simulink model "backup_LQR"  (R2019b)
settings: Solver=ode1  StartTime=0.0  StopTime=Inf  FixedStep=0.001  RelTol=1e-3
PostLoadFcn:
  | , if any(exist('dsrtsu_mdlpostloadfcn', 'file') ~= 0), dsrtsu_mdlpostloadfcn('Execute', bdroot); end,
InitFcn:
  | , if any(exist('rtifpga_mdlclblib', 'file') ~= 0), rtifpga_mdlclblib('Init', bdroot); end,
values from neighbouring files (symbols this model uses):
  ballLQRgain = lqr(ballSystem, Q, R)    [linear_Feedback_ball.m]
  denc_mi = Controller.Denominator{1}    [linear_Feedback_ball.m]
  numc_mi = Controller.Numerator{1}    [linear_Feedback_ball.m]
undefined symbols (not defined in the file or in its folder): Continuous, Time, Ybop0
libraries: rtiemclib x6, rtiethernetlib x3, rti1202lib_dac_class1 x3, ctrlSharedLib x1
(part 1 of 2)
Description:
  | Standard RTI1202 template.
  | Supported MATLAB version:  R2019b.
settings Model: Tag=RTI1202  DSRTSU_INTERNAL_RTI_VER=570  DSRTSU_INTERNAL_RTI_TYPE=rti1202  RTICANMMDATA=struct('GeneralSetupData',struct('modelroot','C:\Users\20200910\Documents\Temp\14062021','generalsettings',struct('filesettings',struct('destfolder',struct('Name','RTICANMM_FILES','Check',1),'buildfolder',struct('Name','.','Check',1),'AbsDestfolder',struct('Name','C:\Users\20200910\Documents\Temp\14062021\RTICANMM_FILES'),'AbsBuildfolder',struct('Name','C:\Users\20200910\Documents\Temp\14062021'))),'options',struct('addpaths',1,'rmpaths',1,'addtrcexclusion',true,'cannavigator',struct('checkmonitoring',0),'show_usrtrc',0,'use_usrtrc',0),'advanced',struct('options',ones(1,100)),'MPSetup',{{}},'RTI',struct('Type','RTI1202','Ver','7.15','Date','02-Nov-2020'),'modelname','backup_LQR','block','backup_LQR'))  DSRTSU_INTERNAL_RTIFPGA=170  Creator=20201603  LastModifiedBy=20200910
settings DataIOCC: ReturnWorkspaceOutputs=off
settings OptimizationCC: BlockReduction=off  OptimizeBlockIOStorage=off  BufferReuse=off  GlobalBufferReuse=off  ExpressionFolding=off  LocalBlockOutputs=off  OptimizeDataStoreBuffers=off  BusAssignmentInplaceUpdate=off
settings DebuggingCC: PregeneratedLibrarySubsystemCodeDiagnostic=none  ArithmeticOperatorsInVariantConditions=warning
settings HardwareCC: ProdBitPerPointer=32  ProdBitPerSizeT=32  ProdBitPerPtrDiffT=32  ProdLargestAtomicInteger=Integer  ProdEndianess=BigEndian  ProdWordSize=32  ProdLongLongMode=on  ProdHWDeviceType=Custom Processor->Custom  TargetIntDivRoundTo=Zero  TargetEndianess=BigEndian  TargetHWDeviceType=Custom Processor->Custom
settings ModelReferenceCC: EnableParallelModelReferenceBuilds=on  ParallelModelReferenceMATLABWorkerInit=Load Top Model
settings SFSimCC: SimUseLocalCustomCode=off  MATLABDynamicMemAlloc=off  CustomCodeUndefinedFunction=UseInterfaceOnly
settings RTWCC: Description=dSPACE DS1202 Hardware Platform  SystemTargetFile=rti1202.tlc  MakeCommand=make_rti  TemplateMakefile=rti1202.tmf  RTWUseLocalCustomCode=off
settings CodeAppCC: StateflowObjectComments=on
settings STFCustomTargetCC: ParMdlRefBuildCompliant=on  SystemTargetFile=rti1202.tlc
settings GRTTargetCC: TargetLangStandard=C89/C90 (ANSI)  CompOptLevelCompliant=off  ConcurrentExecutionCompliant=off  CombineOutputUpdateFcns=off  MatFileLogging=off  CPPClassGenCompliant=off  UseToolchainInfoCompliant=off
settings ConfigComp: CovMetricSettings=dswe

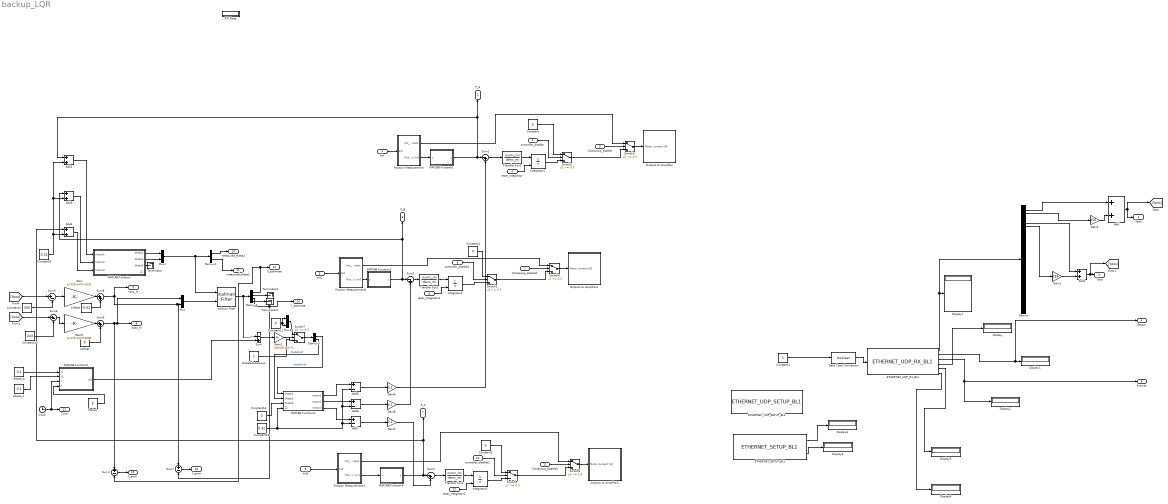
== system backup_LQR ==
  Init : Inport
  controller_disable : Inport  Port=2
  CloseLoop_disable : Inport  Port=3
  reser_integrator : Inport  Port=4
  Init1 : Inport  Port=5
  controller_disable1 : Inport  Port=6
  CloseLoop_disable1 : Inport  Port=7
  reser_integrator1 : Inport  Port=8
  Init2 : Inport  Port=9
  controller_disable2 : Inport  Port=10
  CloseLoop_disable2 : Inport  Port=11
  reser_integrator2 : Inport  Port=12
  Add : Sum  AccumDataTypeStr=uint16
  Add{1..4} (4 alike) : Sum
  Add5 : Sum  Inputs=+-
  Add6 : Sum  Inputs=+-
  Add7 : Sum  Inputs=+-
  Clock : Clock
  Constant{,2..3,11,13} (5 alike) : Constant  Value=0
  Constant1 : Constant
  Constant10 : Constant  Value=243
  Constant14 : Constant  Value=0.32
  Constant4 : Constant  Value=300
  Constant9 : Constant  Value=0.32
  Data Type Conversion : DataTypeConversion  OutDataTypeStr=boolean
  Demux : Demux  Outputs=32
  Demux1 : Demux  Outputs=2
  Demux2 : Demux
  Demux3 : Demux  Outputs=2
  "DisableOuterLoop " : Constant
  Display{,1..7} (8 alike) : Display
      Display7 settings: Format=decimal (Stored Integer)
  ETHERNET_SETUP_BL1 : rtiethernetlib/ETHERNET_SETUP_BL1  DSProperties=struct('RTI',struct('Version',uint32(2),'BlockType',struct('isSLSource',uint8(0),'isSLSink',uint8(0),'isHWSource',uint8(0),'isHWSink',uint8(0),'isSetup',uint8(1),'isInline',uint8(1),'isNonInline',uint8(0),'isInterrupt',uint8(0),'isChannelwise',uint8(0)),'IOBoardType','DSETHERNET','UnitType','ETHERNET','Identifier','SETUP','DialogType','ML','BlockSet','RTIETHERNET','SlaveProcessor','NONE'))  RTIBlockInterface=struct('OutputPortsWidth',int32([3 1 1 4]),'OutputPortsActive',[1 0 0 1],'OutputPortsName',{{['Link Status'],['Watchdog Status'],['DHCP Status'],['Local IP']}},'OutputPortsDataType',{{'SS_UINT32','SS_UINT32','SS_UINT32','SS_UINT8'}},'InitLevel',3,'IconTransparency','on','BlockDisplay',{{['Ethernet Setup\n\nLocal IP: 192.168.141.7'],'left'}},'DialogFcn','rtiethernetsetupgui','BlockName',struct('Token',{{'ETHERNET_SETUP_BL1'}}))  RTIBlockParameters=struct('DHCPserverMode',{{0,'OFF',[0 1]}},'LocalIpNum1',{{'192','OFF',[0 255]}},'LocalIpNum2',{{'168','OFF',[0 255]}},'LocalIpNum3',{{'141','OFF',[0 255]}},'LocalIpNum4',{{'7','OFF',[0 255]}},'SubnetMaskNum1',{{'255','OFF',[0 255]}},'SubnetMaskNum2',{{'255','OFF',[0 255]}},'SubnetMaskNum3',{{'255','OFF',[0 255]}},'SubnetMaskNum4',{{'0','OFF',[0 255]}},'GatewayNum1',{{'0','OFF',[0 255]}},'GatewayNum2',{{'0','OFF',[0 255]}},'GatewayNum3',{{'0','OFF',[0 255]}},'GatewayNum4',{{'0','OFF',[0 255]}},'LinkStatusOutPortMode',{{1,'OFF',[0 1]}},'NumOfEthConnectors',{{3,'ON',[1 16]}},'WatchdogStatusOutPortMode',{{0,'OFF',[0 1]}},'LocalIpOutPortMode',{{1,'OFF',[0 1]}},'IpAndSubmaskCheck',{{int32(1),'OFF',[0 1]}},'TLCFileName',{{'rtiethernetsetup','OFF',[]}})  RTISFcnParameters=struct('DHCPserverMode','int32','LocalIpNum1','uint8','LocalIpNum2','uint8','LocalIpNum3','uint8','LocalIpNum4','uint8','SubnetMaskNum1','uint8','SubnetMaskNum2','uint8','SubnetMaskNum3','uint8','SubnetMaskNum4','uint8','GatewayNum1','uint8','GatewayNum2','uint8','GatewayNum3','uint8','GatewayNum4','uint8','LinkStatusOutPortMode','int32','NumOfEthConnectors','int32','WatchdogStatusOutPortMode','int32','LocalIpOutPortMode','int32','TLCFileName','char')  RTIBlockParaDefault=struct('DHCPserverMode',0,'LocalIpNum1',192,'LocalIpNum2',168,'LocalIpNum3',140,'LocalIpNum4',6,'SubnetMaskNum1',255,'SubnetMaskNum2',255,'SubnetMaskNum3',255,'SubnetMaskNum4',0,'GatewayNum1',0,'GatewayNum2',0,'GatewayNum3',0,'GatewayNum4',0,'LinkStatusOutPortMode',1,'NumOfEthConnectors',3,'WatchdogStatusOutPortMode',0,'LocalIpOutPortMode',0,'IpAndSubmaskCheck',1,'TLCFileName','rtiethernetsetup')
      settings: SourceProductName=dSPACE RTI Ethernet Blockset
  ETHERNET_UDP_RX_BL1 : rtiethernetlib/ETHERNET_UDP_RX_BL1  DSProperties=struct('RTI',struct('Version',uint32(1),'BlockType',struct('isSLSource',uint8(1),'isSLSink',uint8(1),'isHWSource',uint8(0),'isHWSink',uint8(1),'isSetup',uint8(0),'isInline',uint8(1),'isNonInline',uint8(0),'isInterrupt',uint8(0),'isChannelwise',uint8(0)),'IOBoardType','DSETHERNET','UnitType','UDP','Identifier','RXUDP','DialogType','ML','BlockSet','RTIETHERNET','SlaveProcessor','NONE'))  RTIBlockInterface=struct('OutputPortsWidth',int32([32 1 1 1 4 1]),'OutputPortsActive',[1 1 1 1 1 1],'OutputPortsName',{{'Data','Status',['Received Frames'],['Received Bytes'],['Remote IP'],['Remote Port']}},'OutputPortsDataType',{{'SS_UINT8','SS_UINT32','SS_DOUBLE','SS_UINT32','SS_UINT8','SS_UINT16'}},'InputPortsWidth',int32(1),'InputPortsActive',1,'InputPortsName',{{'Enable'}},'InputPortsDataType',{{'SS_BOOLEAN'}},'RWork',{{{'RECEIVED_FRAMES',uint32(1)}}},'InitLevel',3,'IconTransparency','on','BlockDisplay',{{['Ethernet UDP/IP\nRX\n\nSocket ID: 0'],'center'}},'DialogFcn','rtiethernetrxudpgui','BlockName',struct('Token',{{'ETHERNET_UDP_RX_BL1'}}))  RTIBlockParameters=struct('SocketIdIndex',{{2,'OFF',[1 2]}},'SocketId',{{0,'OFF',[-1 inf]}},'RemoteIp',{{['<NOT AVAILABLE>'],'OFF',[]}},'RemotePort',{{['<NOT AVAILABLE>'],'OFF',[]}},'LocalPort',{{49001,'OFF',[]}},'FrameSize',{{'32','OFF',[1 65507]}},'EnableVariableFrameSize',{{1,'OFF',[0 1]}},'VariableFrameSizeMode',{{1,'OFF',[1 2]}},'InterruptMode',{{0,'OFF',[0 1]}},'RemoteIpOutPortMode',{{1,'OFF',[0 1]}},'RemotePortOutPortMode',{{1,'OFF',[0 1]}},'TLCFileName',{{'rtiethernetrxudp','OFF',[]}})  RTISFcnParameters=struct('SocketIdIndex','int32','SocketId','double','FrameSize','uint16','EnableVariableFrameSize','int32','VariableFrameSizeMode','int32','InterruptMode','int32','RemoteIpOutPortMode','int32','RemotePortOutPortMode','int32','TLCFileName','char')  RTIBlockParaDefault=struct('SocketIdIndex',1,'SocketId',-1,'RemoteIp',['<NOT AVAILABLE>'],'RemotePort',['<NOT AVAILABLE>'],'LocalPort',['<NOT AVAILABLE>'],'FrameSize',1024,'EnableVariableFrameSize',0,'VariableFrameSizeMode',1,'InterruptMode',0,'RemoteIpOutPortMode',0,'RemotePortOutPortMode',0,'TLCFileName','rtiethernetrxudp')
      settings: SourceProductName=dSPACE RTI Ethernet Blockset
  ETHERNET_UDP_SETUP_BL1 : rtiethernetlib/ETHERNET_UDP_SETUP_BL1  DSProperties=struct('RTI',struct('Version',uint32(2),'BlockType',struct('isSLSource',uint8(1),'isSLSink',uint8(1),'isHWSource',uint8(0),'isHWSink',uint8(0),'isSetup',uint8(0),'isInline',uint8(1),'isNonInline',uint8(0),'isInterrupt',uint8(0),'isChannelwise',uint8(0)),'IOBoardType','DSETHERNET','UnitType','UDP','Identifier','SETUPUDP','DialogType','ML','BlockSet','RTIETHERNET','SlaveProcessor','NONE'))  RTIBlockInterface=struct('OutputPortsWidth',int32(2),'OutputPortsActive',0,'OutputPortsName',{{['RX Dropped Frames']}},'OutputPortsDataType',{{'SS_DOUBLE'}},'InputPortsWidth',int32([4 1]),'InputPortsActive',int32([0 0]),'InputPortsName',{{['RX Remote IP Filter'],['RX Remote Port Filter']}},'InputPortsDataType',{{'SS_UINT8','SS_UINT16'}},'RWork',{{{'RX_DROPPED_FRAMES',uint32(2)}}},'InitLevel',3,'IconTransparency','on','BlockDisplay',{{['Ethernet UDP/IP\nSetup\n\nSocket ID: 0'],'center'}},'DialogFcn','rtiethernetsetupudpgui','BlockName',struct('Token',{{'ETHERNET_UDP_SETUP_BL1'}}))  RTIBlockParameters=struct('SocketId',{{0,'OFF',[]}},'EnableSocketBind',{{1,'OFF',[0 1]}},'AcceptAnyRxRemoteIp',{{1,'OFF',[0 1]}},'RxRemoteIpNum1',{{'131','OFF',[0 255]}},'RxRemoteIpNum2',{{'155','OFF',[0 255]}},'RxRemoteIpNum3',{{'33','OFF',[0 255]}},'RxRemoteIpNum4',{{'44','OFF',[0 255]}},'EnableDynamicRxRemoteIpFilter',{{0,'OFF',[0 1]}},'AcceptAnyRxRemotePort',{{1,'OFF',[0 1]}},'RxRemotePort',{{'57272','OFF',[1 65535]}},'EnableDynamicRxRemotePortFilter',{{0,'OFF',[0 1]}},'TxRemoteIpNum1',{{'131','OFF',[0 255]}},'TxRemoteIpNum2',{{'155','OFF',[0 255]}},'TxRemoteIpNum3',{{'33','OFF',[0 255]}},'TxRemoteIpNum4',{{'44','OFF',[0 255]}},'TxRemotePort',{{'49002','OFF',[1 65535]}},'SpecifyLocalPort',{{1,'OFF',[0 1]}},'LocalPort',{{'49001','OFF',[1 65535]}},'InterruptMode',{{0,'OFF',[0 1]}},'RxDroppedFramesOutPortMode',{{0,'OFF',[0 1]}},'RemoteIpNumCheck',{{0,'OFF',[0 1]}},'RemotePortCheck',{{0,'OFF',[0 1]}},'LocalPortCheck',{{1,'OFF',[0 1]}},'DHCPserverModeEnabled',{{0,'OFF',[0 1]}},'TLCFileName',{{'rtiethernetsetupudp','OFF',[]}})  RTISFcnParameters=struct('SocketId','double','EnableSocketBind','int32','AcceptAnyRxRemoteIp','int32','RxRemoteIpNum1','uint8','RxRemoteIpNum2','uint8','RxRemoteIpNum3','uint8','RxRemoteIpNum4','uint8','EnableDynamicRxRemoteIpFilter','int32','AcceptAnyRxRemotePort','int32','RxRemotePort','uint16','EnableDynamicRxRemotePortFilter','int32','TxRemoteIpNum1','uint8','TxRemoteIpNum2','uint8','TxRemoteIpNum3','uint8','TxRemoteIpNum4','uint8','TxRemotePort','uint16','SpecifyLocalPort','int32','LocalPort','uint16','InterruptMode','int32','RxDroppedFramesOutPortMode','int32','DHCPserverModeEnabled','int32','TLCFileName','char')  RTIBlockParaDefault=struct('SocketId',-1,'EnableSocketBind',1,'AcceptAnyRxRemoteIp',1,'RxRemoteIpNum1',0,'RxRemoteIpNum2',0,'RxRemoteIpNum3',0,'RxRemoteIpNum4',0,'EnableDynamicRxRemoteIpFilter',0,'AcceptAnyRxRemotePort',1,'RxRemotePort',49002,'EnableDynamicRxRemotePortFilter',0,'TxRemoteIpNum1',0,'TxRemoteIpNum2',0,'TxRemoteIpNum3',0,'TxRemoteIpNum4',0,'TxRemotePort',49002,'SpecifyLocalPort',0,'LocalPort',49001,'InterruptMode',0,'RxDroppedFramesOutPortMode',0,'RemoteIpNumCheck',0,'RemotePortCheck',0,'LocalPortCheck',0,'DHCPserverModeEnabled',0,'TLCFileName','rtiethernetsetupudp')
      settings: SourceProductName=dSPACE RTI Ethernet Blockset
  Gain : Gain  Gain=1/(536-54)*0.3595
  Gain1 : Gain  Gain=256  OutDataTypeStr=uint16
  Gain2 : Gain  Gain=256  OutDataTypeStr=uint16
  Gain3 : Gain  Gain=ballLQRgain  Multiplication=Matrix(K*u)
  Gain5 : Gain  Gain=1/(475-14)*0.3595
  GainA : Gain  Gain=0.1
  GainB : Gain  Gain=0.1
  GainC : Gain  Gain=0.1
  Integrator1 : Integrator  ExternalReset=rising  LimitOutput=on  UpperSaturationLimit=3  LowerSaturationLimit=-3
  Integrator2 : Integrator  ExternalReset=rising  LimitOutput=on  UpperSaturationLimit=3  LowerSaturationLimit=-3
  Integrator3 : Integrator  ExternalReset=rising  LimitOutput=on  UpperSaturationLimit=3  LowerSaturationLimit=-3
  Kalman Filter : ctrlSharedLib/Kalman Filter  TimeDomain=Continuous-Time  UseCurrentEstimator=on  ModelSource=LTI State-Space Variable  ModelSourceVariable=ballSystem  A=0.95  B=1  C=1  D=0  NumberOfStates=1  NumberOfInputs=1  NumberOfOutputs=1  InitialEstimateSource=Dialog  X0=Ybop0  P0=10  UseK=off  UseGH=off  NumberOfProcessNoiseInputs=1  G=1  TimeInvariantG=on  H=0  TimeInvariantH=on  Q=diag([1 20 1 20])  TimeInvariantQ=on  R=diag([0.01 0.01])  TimeInvariantR=on  N=0  TimeInvariantN=on  AddInputPort=on  AddEnablePort=off  OutputEstimatedY=off  OutputP=off  Ts=-1
      settings: SourceProductBaseCode=CT
  MATLAB Function : MATLAB Function  TreatAsAtomicUnit=on
  MATLAB Function1 : MATLAB Function  TreatAsAtomicUnit=on
  MATLAB Function2 : MATLAB Function  TreatAsAtomicUnit=on
  MATLAB Function3 : MATLAB Function  TreatAsAtomicUnit=on
  MATLAB Function4 : MATLAB Function  TreatAsAtomicUnit=on
  MATLAB Function5 : MATLAB Function  TreatAsAtomicUnit=on
  Mux : Mux  Inputs=2
  Mux1 : Mux  Inputs=2
  Mux4 : Mux  Inputs=2
  Outputs to Amplifier : Subsystem  TreatAsAtomicUnit=on
  Outputs to Amplifier1 : Subsystem  TreatAsAtomicUnit=on
  Outputs to Amplifier2 : Subsystem  TreatAsAtomicUnit=on
  Period : Constant  Value=5
  Position Measurement : Subsystem  TreatAsAtomicUnit=on
  Position Measurement1 : Subsystem  TreatAsAtomicUnit=on
  Position Measurement2 : Subsystem  TreatAsAtomicUnit=on
  RTI Data : Subsystem  Tag=struct('RTIDataServer',struct('RTIDataServerVs','2','RTIModelDescription','struct(''main'',''backup_LQR'',''sub'','''',''isMp'',0)'))  LoadFcn="if exist('rtidc'), try,  rtidc('DataHostBlockClbLoad', gcbh); catch, disp(['Warning: ''LoadFcn'' for RTI Data block failed: ' lasterr]); end, end,"  mask(RTI_DATA_HOST){}
      mask help:
      | RTI Data Block.
      | This block is used by RTI to store internal model-dependent data.
      | Please keep this block on the root level of the model. Deleting this block will result in data loss.
      |
      | NEVER DELETE OR COPY THIS BLOCK!
      settings: CopyFcn="if exist('rtidc'), try,  rtidc('DataHostBlockClbCopy', gcbh); catch, disp(['Warning: ''CopyFcn'' for RTI Data block failed: ' lasterr]); end, end,"  DeleteFcn="if exist('rtidc'), try,  rtidc('DataHostBlockClbDelete', gcbh); catch, disp(['Warning: ''DeleteFcn'' for RTI Data block failed: ' lasterr]); end, end,"  ModelCloseFcn="if exist('rtidc'), try,  rtidc('DataHostBlockClbModelClose', gcbh); catch, disp(['Warning: ''ModelCloseFcn'' for RTI Data block failed: ' lasterr]); end, end,"  PreSaveFcn="if exist('rtidc'), try,  rtidc('DataHostBlockClbPreSave', gcbh); catch, disp(['Warning: ''PreSaveFcn'' for RTI Data block failed: ' lasterr]); end, end,"  PostSaveFcn="if exist('rtidc'), try,  rtidc('DataHostBlockClbPostSave', gcbh); catch, disp(['Warning: ''PostSaveFcn'' for RTI Data block failed: ' lasterr]); end, end,"  NameChangeFcn="if exist('rtidc'), try,  rtidc('DataHostBlockClbNameChange', gcbh); catch, disp(['Warning: ''NameChangeFcn'' for RTI Data block failed: ' lasterr]); end, end,"
      mask Help:
      | RTI Data Block.
      | This block is used by RTI to store internal model-dependent data.
      | Please keep this block on the root level of the model. Deleting this block will result in data loss.
      | 
      | NEVER DELETE OR COPY THIS BLOCK!
      mask Display:
      | text(0.5, 0.5, 'RTI Data', 'HorizontalAlignment', 'center');
      | plot([1 0]);
  Sum : Sum  Inputs=|-+
  Sum1 : Sum  Inputs=|-+  SaturateOnIntegerOverflow=on
  Sum2 : Sum  Inputs=|-+  SaturateOnIntegerOverflow=on
  Sum3 : Sum  Inputs=|-+  SaturateOnIntegerOverflow=on
  Sum4 : Sum  Inputs=+-
  Sum5 : Sum  Inputs=|+-
  Sum6 : Sum  Inputs=|+-
  Sum7 : Sum  Inputs=+-
  Sum8 : Sum  Inputs=|++
  Sum9 : Sum  Inputs=|++
  Switch{1..7} (7 alike) : Switch  Threshold=0.5
  Terminator : Terminator
  Terminator1 : Terminator
  Terminator2 : Terminator
  Transfer Fcn1 : TransferFcn  Numerator=numc_mi  Denominator=denc_mi
  Transfer Fcn2 : TransferFcn  Numerator=numc_mi  Denominator=denc_mi
  Transfer Fcn3 : TransferFcn  Numerator=numc_mi  Denominator=denc_mi
  Xoffset : Constant  Value=0
  Yoffset : Constant  Value=-0.02
  ellipse_a : Constant  Value=0.1
  ellipse_b : Constant  Value=0.1
  P_A : Outport
  "Xpos " : Outport  Port=2
  "Ypos " : Outport  Port=3
  "Status " : Outport  Port=4
  "Frames " : Outport  Port=5
  P_B : Outport  Port=6
  P_C : Outport  Port=7
  Xpos_m : Outport  Port=8
  Ypos_m : Outport  Port=9
  measured_theta1 : Outport  Port=10
  measured_theta2 : Outport  Port=11
  Time : Outport  Port=12
  X_estimate : Outport  Port=13
  Y_estimate : Outport  Port=14
  X_error : Outport  Port=15
  Y_error : Outport  Port=16
  wires:
  Add5/1 -> GainA/1
  reser_integrator/1 -> Integrator2/2
  controller_disable/1 -> Switch2/2
  CloseLoop_disable/1 -> Switch3/2
  Position Measurement/1(init_current) -> Switch3/1
  Init/1 -> Position Measurement/1(Init)
  Constant/1 -> Switch2/1
  Switch3/1 -> Outputs to Amplifier/1(Motor current [A])
  Switch2/1 -> Switch3/3
  Gain2/1 -> Add/2
  Demux/1 -> Add/1
  Add1/1 -> [Ypos], "Ypos "/1
  ETHERNET_SETUP_BL1/2 -> Display3/1
  Demux/2 -> Gain2/1
  ETHERNET_UDP_RX_BL1/2 -> "Status "/1, Display1/1
  ETHERNET_UDP_RX_BL1/6 -> Display4/1
  Demux/5 -> Add1/1
  ETHERNET_UDP_RX_BL1/4 -> Display/1
  Data Type Conversion/1 -> ETHERNET_UDP_RX_BL1/1
  ETHERNET_UDP_RX_BL1/3 -> "Frames "/1, Display2/1
  Constant1/1 -> Data Type Conversion/1
  Add/1 -> "Xpos "/1, [Xpos]
  Gain1/1 -> Add1/2
  Demux/6 -> Gain1/1
  ETHERNET_SETUP_BL1/1 -> Display6/1
  ETHERNET_UDP_RX_BL1/1 -> Display7/1, Demux/1
  ETHERNET_UDP_RX_BL1/5 -> Display5/1
  CloseLoop_disable1/1 -> Switch4/2
  Init1/1 -> Position Measurement1/1(Init)
  Add6/1 -> GainB/1
  controller_disable1/1 -> Switch1/2
  reser_integrator1/1 -> Integrator1/2
  MATLAB Function2/1(y) -> Add3/1, P_B/1, Sum2/1
  Switch4/1 -> Outputs to Amplifier1/1(Motor current [A])
  Constant2/1 -> Switch1/1
  Position Measurement1/1(init_current) -> Switch4/1
  Switch1/1 -> Switch4/3
  Constant3/1 -> Switch5/1
  controller_disable2/1 -> Switch5/2
  CloseLoop_disable2/1 -> Switch6/2
  Init2/1 -> Position Measurement2/1(Init)
  reser_integrator2/1 -> Integrator3/2
  Position Measurement2/1(init_current) -> Switch6/1
  Switch6/1 -> Outputs to Amplifier2/1(Motor current [A])
  Switch5/1 -> Switch6/3
  MATLAB Function4/1(y) -> P_C/1, Add4/1, Sum3/1
  Sum6/1 -> Gain5/1
  MATLAB Function1/1(y) -> P_A/1, Add2/1, Sum1/1
  Sum5/1 -> Gain/1
  MATLAB Function/3(theta3) -> Terminator/1
  Constant10/1 -> Sum6/2
  Add2/1 -> MATLAB Function/1(motor1)
  MATLAB Function/1(theta1) -> Mux1/1
  Constant9/1 -> Add4/2, Add3/2, Add2/2
  Add3/1 -> MATLAB Function/2(motor2)
  Constant4/1 -> Sum5/2
  Sum8/1 -> Sum7/1, Mux/2, Ypos_m/1
  [Xpos] -> Sum5/1
  Add4/1 -> MATLAB Function/3(motor3)
  [Ypos] -> Sum6/1
  MATLAB Function/2(theta2) -> Mux1/2
  Constant13/1 -> MATLAB Function3/3(theta3)
  MATLAB Function3/1(motor1) -> Add5/1
  MATLAB Function3/2(motor2) -> Add6/1
  MATLAB Function3/3(motor3) -> Add7/1
  Constant14/1 -> MATLAB Function3/4(Zc), Add7/2, Add6/2, Add5/2
  GainA/1 -> Sum1/2
  GainB/1 -> Sum2/2
  Add7/1 -> GainC/1
  Mux1/1 -> Kalman Filter/1, Demux1/1
  Demux3/1 -> MATLAB Function3/1(theta1)  "theta1ref"
  Demux3/2 -> MATLAB Function3/2(theta2)  "theta2ref"
  MATLAB Function5/1(ref) -> Sum/2
  Kalman Filter/1 -> Sum/1, Demux2/1
  Sum/1 -> Gain3/1
  Mux/1 -> Kalman Filter/2
  Demux1/1 -> measured_theta1/1
  Demux1/2 -> measured_theta2/1
  Position Measurement/2(Position [m]) -> MATLAB Function1/1(u)
  Position Measurement1/2(Position [m]) -> MATLAB Function2/1(u)
  Position Measurement2/2(Position [m]) -> MATLAB Function4/1(u)
  Sum9/1 -> Xpos_m/1, Mux/1, Sum4/1
  Integrator2/1 -> Switch2/3
  Integrator1/1 -> Switch1/3
  Integrator3/1 -> Switch5/3
  Sum3/1 -> Transfer Fcn3/1
  Sum2/1 -> Transfer Fcn1/1
  Transfer Fcn1/1 -> Integrator1/1
  Sum1/1 -> Transfer Fcn2/1
  Transfer Fcn2/1 -> Integrator2/1
  Transfer Fcn3/1 -> Integrator3/1
  Constant11/1 -> Mux4/1, Mux4/2
  Mux4/1 -> Switch7/1
  "DisableOuterLoop "/1 -> Switch7/2
  Gain3/1 -> Switch7/3
  Switch7/1 -> Demux3/1
  GainC/1 -> Sum3/2
  Clock/1 -> MATLAB Function5/3(t), Time/1
  Demux2/1 -> X_estimate/1, Sum4/2
  Demux2/3 -> Sum7/2, Y_estimate/1
  Demux2/2 -> Terminator1/1
  Demux2/4 -> Terminator2/1
  Sum4/1 -> X_error/1
  Sum7/1 -> Y_error/1
  ellipse_a/1 -> MATLAB Function5/1(r1)
  ellipse_b/1 -> MATLAB Function5/2(r2)
  Period/1 -> MATLAB Function5/4(T)
  Gain/1 -> Sum8/1
  Yoffset/1 -> Sum8/2
  Gain5/1 -> Sum9/1
  Xoffset/1 -> Sum9/2

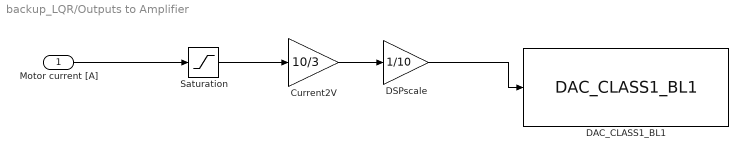
== system backup_LQR/Outputs to Amplifier ==
  Motor current [A] : Inport
  Current2V : Gain  Gain=10/3  SaturateOnIntegerOverflow=on  OutDataTypeStr=Inherit: Same as input  ParamDataTypeStr=Inherit: Same as input
  DAC_CLASS1_BL1 : rti1202lib_dac_class1/DAC_CLASS1_BL1  DSProperties=struct('RTI',struct('Version',uint32(2),'BlockType',struct('isSLSource',uint8(0),'isSLSink',uint8(1),'isHWSource',uint8(0),'isHWSink',uint8(1),'isSetup',uint8(0),'isInline',uint8(1),'isNonInline',uint8(0),'isInterrupt',uint8(0),'isChannelwise',uint8(1)),'IOBoardType',{{'DS120X','STD','DACC1'}},'UnitType','DAC','Identifier','DAC','DialogType','ML','BlockSet','NONE','SlaveProcessor','NONE'))  RTIBlockInterface=struct('InputPortsActive',1,'InputPortsWidth',int32(1),'InputPortsDataType',{{'SS_DOUBLE'}},'InputPortsName',{{['DAC 1']}},'DialogFcn','rti120xstddacc1dacgui','InitLevel',3,'IconTransparency','on','BlockDisplay',{{['DAC CL1\nChannel: 1'],'center'}},'BlockName',struct('Token',{{'DAC_CLASS1_BL1'}}))  RTIBlockParameters=struct('ChannelNo',{{1,'OFF',[]}},'ChannelNumOf',{{1,'OFF',[]}},'InitialValue1',{{'0','OFF',[-10 10]}},'InitialValue2',{{'0','OFF',[-10 10]}},'InitialValue3',{{'0','OFF',[-10 10]}},'InitialValue4',{{'0','OFF',[-10 10]}},'InitialValue5',{{'0','OFF',[-10 10]}},'InitialValue6',{{'0','OFF',[-10 10]}},'InitialValue7',{{'0','OFF',[-10 10]}},'InitialValue8',{{'0','OFF',[-10 10]}},'InitialValue9',{{'0','OFF',[-10 10]}},'InitialValue10',{{'0','OFF',[-10 10]}},'InitialValue11',{{'0','OFF',[-10 10]}},'InitialValue12',{{'0','OFF',[-10 10]}},'InitialValue13',{{'0','OFF',[-10 10]}},'InitialValue14',{{'0','OFF',[-10 10]}},'InitialValue15',{{'0','OFF',[-10 10]}},'InitialValue16',{{'0','OFF',[-10 10]}},'OutputMode',{{ones(1,16),'OFF',[1 2]}},'TermValue1',{{'0','OFF',[-10 10]}},'TermValue2',{{'0','OFF',[-10 10]}},'TermValue3',{{'0','OFF',[-10 10]}},'TermValue4',{{'0','OFF',[-10 10]}},'TermValue5',{{'0','OFF',[-10 10]}},'TermValue6',{{'0','OFF',[-10 10]}},'TermValue7',{{'0','OFF',[-10 10]}},'TermValue8',{{'0','OFF',[-10 10]}},'TermValue9',{{'0','OFF',[-10 10]}},'TermValue10',{{'0','OFF',[-10 10]}},'TermValue11',{{'0','OFF',[-10 10]}},'TermValue12',{{'0','OFF',[-10 10]}},'TermValue13',{{'0','OFF',[-10 10]}},'TermValue14',{{'0','OFF',[-10 10]}},'TermValue15',{{'0','OFF',[-10 10]}},'TermValue16',{{'0','OFF',[-10 10]}},'EnableTermMode',{{0,'OFF',[0 1]}},'TLCFileName',{{'rti120xdac_c1_dac','OFF',[]}},'InitialValueBuildCheck1',{{1,'OFF',[]}},'InitialValueBuildCheck2',{{0,'OFF',[]}},'InitialValueBuildCheck3',{{0,'OFF',[]}},'InitialValueBuildCheck4',{{0,'OFF',[]}},'InitialValueBuildCheck5',{{0,'OFF',[]}},'InitialValueBuildCheck6',{{0,'OFF',[]}},'InitialValueBuildCheck7',{{0,'OFF',[]}},'InitialValueBuildCheck8',{{0,'OFF',[]}},'InitialValueBuildCheck9',{{0,'OFF',[]}},'InitialValueBuildCheck10',{{0,'OFF',[]}},'InitialValueBuildCheck11',{{0,'OFF',[]}},'InitialValueBuildCheck12',{{0,'OFF',[]}},'InitialValueBuildCheck13',{{0,'OFF',[]}},'InitialValueBuildCheck14',{{0,'OFF',[]}},'InitialValueBuildCheck15',{{0,'OFF',[]}},'InitialValueBuildCheck16',{{0,'OFF',[]}},'TermValueBuildCheck1',{{0,'OFF',[]}},'TermValueBuildCheck2',{{0,'OFF',[]}},'TermValueBuildCheck3',{{0,'OFF',[]}},'TermValueBuildCheck4',{{0,'OFF',[]}},'TermValueBuildCheck5',{{0,'OFF',[]}},'TermValueBuildCheck6',{{0,'OFF',[]}},'TermValueBuildCheck7',{{0,'OFF',[]}},'TermValueBuildCheck8',{{0,'OFF',[]}},'TermValueBuildCheck9',{{0,'OFF',[]}},'TermValueBuildCheck10',{{0,'OFF',[]}},'TermValueBuildCheck11',{{0,'OFF',[]}},'TermValueBuildCheck12',{{0,'OFF',[]}},'TermValueBuildCheck13',{{0,'OFF',[]}},'TermValueBuildCheck14',{{0,'OFF',[]}},'TermValueBuildCheck15',{{0,'OFF',[]}},'TermValueBuildCheck16',{{0,'OFF',[]}})  RTISFcnParameters=struct('ChannelNo','int16','ChannelNumOf','int16','InitialValue1','double','InitialValue2','double','InitialValue3','double','InitialValue4','double','InitialValue5','double','InitialValue6','double','InitialValue7','double','InitialValue8','double','InitialValue9','double','InitialValue10','double','InitialValue11','double','InitialValue12','double','InitialValue13','double','InitialValue14','double','InitialValue15','double','InitialValue16','double','OutputMode','int16','TermValue1','double','TermValue2','double','TermValue3','double','TermValue4','double','TermValue5','double','TermValue6','double','TermValue7','double','TermValue8','double','TermValue9','double','TermValue10','double','TermValue11','double','TermValue12','double','TermValue13','double','TermValue14','double','TermValue15','double','TermValue16','double','EnableTermMode','int16','TLCFileName','char')  RTIBlockParaDefault=struct('ChannelNo',1,'ChannelNumOf',1,'InitialValue1',0,'InitialValue2',0,'InitialValue3',0,'InitialValue4',0,'InitialValue5',0,'InitialValue6',0,'InitialValue7',0,'InitialValue8',0,'InitialValue9',0,'InitialValue10',0,'InitialValue11',0,'InitialValue12',0,'InitialValue13',0,'InitialValue14',0,'InitialValue15',0,'InitialValue16',0,'OutputMode',ones(1,16),'TermValue1',0,'TermValue2',0,'TermValue3',0,'TermValue4',0,'TermValue5',0,'TermValue6',0,'TermValue7',0,'TermValue8',0,'TermValue9',0,'TermValue10',0,'TermValue11',0,'TermValue12',0,'TermValue13',0,'TermValue14',0,'TermValue15',0,'TermValue16',0,'EnableTermMode',0,'TLCFileName','rti120xdac_c1_dac','InitialValueBuildCheck1',0,'InitialValueBuildCheck2',0,'InitialValueBuildCheck3',0,'InitialValueBuildCheck4',0,'InitialValueBuildCheck5',0,'InitialValueBuildCheck6',0,'InitialValueBuildCheck7',0,'InitialValueBuildCheck8',0,'InitialValueBuildCheck9',0,'InitialValueBuildCheck10',0,'InitialValueBuildCheck11',0,'InitialValueBuildCheck12',0,'InitialValueBuildCheck13',0,'InitialValueBuildCheck14',0,'InitialValueBuildCheck15',0,'InitialValueBuildCheck16',0,'TermValueBuildCheck1',0,'TermValueBuildCheck2',0,'TermValueBuildCheck3',0,'TermValueBuildCheck4',0,'TermValueBuildCheck5',0,'TermValueBuildCheck6',0,'TermValueBuildCheck7',0,'TermValueBuildCheck8',0,'TermValueBuildCheck9',0,'TermValueBuildCheck10',0,'TermValueBuildCheck11',0,'TermValueBuildCheck12',0,'TermValueBuildCheck13',0,'TermValueBuildCheck14',0,'TermValueBuildCheck15',0,'TermValueBuildCheck16',0)
  DSPscale : Gain  Gain=1/10  SaturateOnIntegerOverflow=on  OutDataTypeStr=Inherit: Same as input  ParamDataTypeStr=Inherit: Same as input
  Saturation : Saturate  UpperLimit=3  LowerLimit=-3
  wires:
  Saturation/1 -> Current2V/1
  Current2V/1 -> DSPscale/1
  Motor current [A]/1 -> Saturation/1
  DSPscale/1 -> DAC_CLASS1_BL1/1

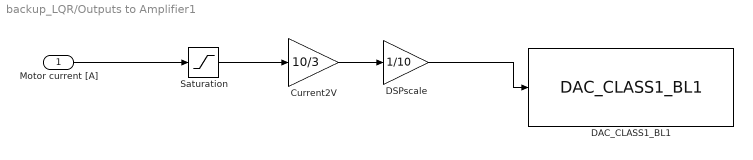
== system backup_LQR/Outputs to Amplifier1 ==
  Motor current [A] : Inport
  Current2V : Gain  Gain=10/3  SaturateOnIntegerOverflow=on  OutDataTypeStr=Inherit: Same as input  ParamDataTypeStr=Inherit: Same as input
  DAC_CLASS1_BL1 : rti1202lib_dac_class1/DAC_CLASS1_BL1  DSProperties=struct('RTI',struct('Version',uint32(2),'BlockType',struct('isSLSource',uint8(0),'isSLSink',uint8(1),'isHWSource',uint8(0),'isHWSink',uint8(1),'isSetup',uint8(0),'isInline',uint8(1),'isNonInline',uint8(0),'isInterrupt',uint8(0),'isChannelwise',uint8(1)),'IOBoardType',{{'DS120X','STD','DACC1'}},'UnitType','DAC','Identifier','DAC','DialogType','ML','BlockSet','NONE','SlaveProcessor','NONE'))  RTIBlockInterface=struct('InputPortsActive',1,'InputPortsWidth',int32(1),'InputPortsDataType',{{'SS_DOUBLE'}},'InputPortsName',{{['DAC 2']}},'DialogFcn','rti120xstddacc1dacgui','InitLevel',3,'IconTransparency','on','BlockDisplay',{{['DAC CL1\nChannel: 2'],'center'}},'BlockName',struct('Token',{{'DAC_CLASS1_BL1'}}))  RTIBlockParameters=struct('ChannelNo',{{2,'OFF',[]}},'ChannelNumOf',{{1,'OFF',[]}},'InitialValue1',{{'0','OFF',[-10 10]}},'InitialValue2',{{'0','OFF',[-10 10]}},'InitialValue3',{{'0','OFF',[-10 10]}},'InitialValue4',{{'0','OFF',[-10 10]}},'InitialValue5',{{'0','OFF',[-10 10]}},'InitialValue6',{{'0','OFF',[-10 10]}},'InitialValue7',{{'0','OFF',[-10 10]}},'InitialValue8',{{'0','OFF',[-10 10]}},'InitialValue9',{{'0','OFF',[-10 10]}},'InitialValue10',{{'0','OFF',[-10 10]}},'InitialValue11',{{'0','OFF',[-10 10]}},'InitialValue12',{{'0','OFF',[-10 10]}},'InitialValue13',{{'0','OFF',[-10 10]}},'InitialValue14',{{'0','OFF',[-10 10]}},'InitialValue15',{{'0','OFF',[-10 10]}},'InitialValue16',{{'0','OFF',[-10 10]}},'OutputMode',{{ones(1,16),'OFF',[1 2]}},'TermValue1',{{'0','OFF',[-10 10]}},'TermValue2',{{'0','OFF',[-10 10]}},'TermValue3',{{'0','OFF',[-10 10]}},'TermValue4',{{'0','OFF',[-10 10]}},'TermValue5',{{'0','OFF',[-10 10]}},'TermValue6',{{'0','OFF',[-10 10]}},'TermValue7',{{'0','OFF',[-10 10]}},'TermValue8',{{'0','OFF',[-10 10]}},'TermValue9',{{'0','OFF',[-10 10]}},'TermValue10',{{'0','OFF',[-10 10]}},'TermValue11',{{'0','OFF',[-10 10]}},'TermValue12',{{'0','OFF',[-10 10]}},'TermValue13',{{'0','OFF',[-10 10]}},'TermValue14',{{'0','OFF',[-10 10]}},'TermValue15',{{'0','OFF',[-10 10]}},'TermValue16',{{'0','OFF',[-10 10]}},'EnableTermMode',{{0,'OFF',[0 1]}},'TLCFileName',{{'rti120xdac_c1_dac','OFF',[]}},'InitialValueBuildCheck1',{{0,'OFF',[]}},'InitialValueBuildCheck2',{{1,'OFF',[]}},'InitialValueBuildCheck3',{{0,'OFF',[]}},'InitialValueBuildCheck4',{{0,'OFF',[]}},'InitialValueBuildCheck5',{{0,'OFF',[]}},'InitialValueBuildCheck6',{{0,'OFF',[]}},'InitialValueBuildCheck7',{{0,'OFF',[]}},'InitialValueBuildCheck8',{{0,'OFF',[]}},'InitialValueBuildCheck9',{{0,'OFF',[]}},'InitialValueBuildCheck10',{{0,'OFF',[]}},'InitialValueBuildCheck11',{{0,'OFF',[]}},'InitialValueBuildCheck12',{{0,'OFF',[]}},'InitialValueBuildCheck13',{{0,'OFF',[]}},'InitialValueBuildCheck14',{{0,'OFF',[]}},'InitialValueBuildCheck15',{{0,'OFF',[]}},'InitialValueBuildCheck16',{{0,'OFF',[]}},'TermValueBuildCheck1',{{0,'OFF',[]}},'TermValueBuildCheck2',{{0,'OFF',[]}},'TermValueBuildCheck3',{{0,'OFF',[]}},'TermValueBuildCheck4',{{0,'OFF',[]}},'TermValueBuildCheck5',{{0,'OFF',[]}},'TermValueBuildCheck6',{{0,'OFF',[]}},'TermValueBuildCheck7',{{0,'OFF',[]}},'TermValueBuildCheck8',{{0,'OFF',[]}},'TermValueBuildCheck9',{{0,'OFF',[]}},'TermValueBuildCheck10',{{0,'OFF',[]}},'TermValueBuildCheck11',{{0,'OFF',[]}},'TermValueBuildCheck12',{{0,'OFF',[]}},'TermValueBuildCheck13',{{0,'OFF',[]}},'TermValueBuildCheck14',{{0,'OFF',[]}},'TermValueBuildCheck15',{{0,'OFF',[]}},'TermValueBuildCheck16',{{0,'OFF',[]}})  RTISFcnParameters=struct('ChannelNo','int16','ChannelNumOf','int16','InitialValue1','double','InitialValue2','double','InitialValue3','double','InitialValue4','double','InitialValue5','double','InitialValue6','double','InitialValue7','double','InitialValue8','double','InitialValue9','double','InitialValue10','double','InitialValue11','double','InitialValue12','double','InitialValue13','double','InitialValue14','double','InitialValue15','double','InitialValue16','double','OutputMode','int16','TermValue1','double','TermValue2','double','TermValue3','double','TermValue4','double','TermValue5','double','TermValue6','double','TermValue7','double','TermValue8','double','TermValue9','double','TermValue10','double','TermValue11','double','TermValue12','double','TermValue13','double','TermValue14','double','TermValue15','double','TermValue16','double','EnableTermMode','int16','TLCFileName','char')  RTIBlockParaDefault=struct('ChannelNo',1,'ChannelNumOf',1,'InitialValue1',0,'InitialValue2',0,'InitialValue3',0,'InitialValue4',0,'InitialValue5',0,'InitialValue6',0,'InitialValue7',0,'InitialValue8',0,'InitialValue9',0,'InitialValue10',0,'InitialValue11',0,'InitialValue12',0,'InitialValue13',0,'InitialValue14',0,'InitialValue15',0,'InitialValue16',0,'OutputMode',ones(1,16),'TermValue1',0,'TermValue2',0,'TermValue3',0,'TermValue4',0,'TermValue5',0,'TermValue6',0,'TermValue7',0,'TermValue8',0,'TermValue9',0,'TermValue10',0,'TermValue11',0,'TermValue12',0,'TermValue13',0,'TermValue14',0,'TermValue15',0,'TermValue16',0,'EnableTermMode',0,'TLCFileName','rti120xdac_c1_dac','InitialValueBuildCheck1',0,'InitialValueBuildCheck2',0,'InitialValueBuildCheck3',0,'InitialValueBuildCheck4',0,'InitialValueBuildCheck5',0,'InitialValueBuildCheck6',0,'InitialValueBuildCheck7',0,'InitialValueBuildCheck8',0,'InitialValueBuildCheck9',0,'InitialValueBuildCheck10',0,'InitialValueBuildCheck11',0,'InitialValueBuildCheck12',0,'InitialValueBuildCheck13',0,'InitialValueBuildCheck14',0,'InitialValueBuildCheck15',0,'InitialValueBuildCheck16',0,'TermValueBuildCheck1',0,'TermValueBuildCheck2',0,'TermValueBuildCheck3',0,'TermValueBuildCheck4',0,'TermValueBuildCheck5',0,'TermValueBuildCheck6',0,'TermValueBuildCheck7',0,'TermValueBuildCheck8',0,'TermValueBuildCheck9',0,'TermValueBuildCheck10',0,'TermValueBuildCheck11',0,'TermValueBuildCheck12',0,'TermValueBuildCheck13',0,'TermValueBuildCheck14',0,'TermValueBuildCheck15',0,'TermValueBuildCheck16',0)
  DSPscale : Gain  Gain=1/10  SaturateOnIntegerOverflow=on  OutDataTypeStr=Inherit: Same as input  ParamDataTypeStr=Inherit: Same as input
  Saturation : Saturate  UpperLimit=3  LowerLimit=-3
  wires:
  Saturation/1 -> Current2V/1
  Current2V/1 -> DSPscale/1
  Motor current [A]/1 -> Saturation/1
  DSPscale/1 -> DAC_CLASS1_BL1/1

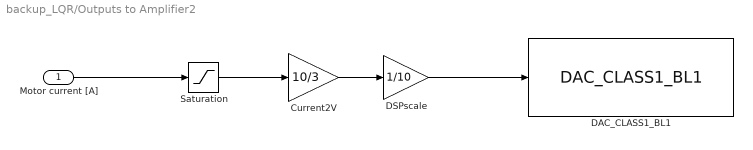
== system backup_LQR/Outputs to Amplifier2 ==
  Motor current [A] : Inport
  Current2V : Gain  Gain=10/3  SaturateOnIntegerOverflow=on  OutDataTypeStr=Inherit: Same as input  ParamDataTypeStr=Inherit: Same as input
  DAC_CLASS1_BL1 : rti1202lib_dac_class1/DAC_CLASS1_BL1  DSProperties=struct('RTI',struct('Version',uint32(2),'BlockType',struct('isSLSource',uint8(0),'isSLSink',uint8(1),'isHWSource',uint8(0),'isHWSink',uint8(1),'isSetup',uint8(0),'isInline',uint8(1),'isNonInline',uint8(0),'isInterrupt',uint8(0),'isChannelwise',uint8(1)),'IOBoardType',{{'DS120X','STD','DACC1'}},'UnitType','DAC','Identifier','DAC','DialogType','ML','BlockSet','NONE','SlaveProcessor','NONE'))  RTIBlockInterface=struct('InputPortsActive',1,'InputPortsWidth',int32(1),'InputPortsDataType',{{'SS_DOUBLE'}},'InputPortsName',{{['DAC 3']}},'DialogFcn','rti120xstddacc1dacgui','InitLevel',3,'IconTransparency','on','BlockDisplay',{{['DAC CL1\nChannel: 3'],'center'}},'BlockName',struct('Token',{{'DAC_CLASS1_BL1'}}))  RTIBlockParameters=struct('ChannelNo',{{3,'OFF',[]}},'ChannelNumOf',{{1,'OFF',[]}},'InitialValue1',{{'0','OFF',[-10 10]}},'InitialValue2',{{'0','OFF',[-10 10]}},'InitialValue3',{{'0','OFF',[-10 10]}},'InitialValue4',{{'0','OFF',[-10 10]}},'InitialValue5',{{'0','OFF',[-10 10]}},'InitialValue6',{{'0','OFF',[-10 10]}},'InitialValue7',{{'0','OFF',[-10 10]}},'InitialValue8',{{'0','OFF',[-10 10]}},'InitialValue9',{{'0','OFF',[-10 10]}},'InitialValue10',{{'0','OFF',[-10 10]}},'InitialValue11',{{'0','OFF',[-10 10]}},'InitialValue12',{{'0','OFF',[-10 10]}},'InitialValue13',{{'0','OFF',[-10 10]}},'InitialValue14',{{'0','OFF',[-10 10]}},'InitialValue15',{{'0','OFF',[-10 10]}},'InitialValue16',{{'0','OFF',[-10 10]}},'OutputMode',{{ones(1,16),'OFF',[1 2]}},'TermValue1',{{'0','OFF',[-10 10]}},'TermValue2',{{'0','OFF',[-10 10]}},'TermValue3',{{'0','OFF',[-10 10]}},'TermValue4',{{'0','OFF',[-10 10]}},'TermValue5',{{'0','OFF',[-10 10]}},'TermValue6',{{'0','OFF',[-10 10]}},'TermValue7',{{'0','OFF',[-10 10]}},'TermValue8',{{'0','OFF',[-10 10]}},'TermValue9',{{'0','OFF',[-10 10]}},'TermValue10',{{'0','OFF',[-10 10]}},'TermValue11',{{'0','OFF',[-10 10]}},'TermValue12',{{'0','OFF',[-10 10]}},'TermValue13',{{'0','OFF',[-10 10]}},'TermValue14',{{'0','OFF',[-10 10]}},'TermValue15',{{'0','OFF',[-10 10]}},'TermValue16',{{'0','OFF',[-10 10]}},'EnableTermMode',{{0,'OFF',[0 1]}},'TLCFileName',{{'rti120xdac_c1_dac','OFF',[]}},'InitialValueBuildCheck1',{{0,'OFF',[]}},'InitialValueBuildCheck2',{{0,'OFF',[]}},'InitialValueBuildCheck3',{{1,'OFF',[]}},'InitialValueBuildCheck4',{{0,'OFF',[]}},'InitialValueBuildCheck5',{{0,'OFF',[]}},'InitialValueBuildCheck6',{{0,'OFF',[]}},'InitialValueBuildCheck7',{{0,'OFF',[]}},'InitialValueBuildCheck8',{{0,'OFF',[]}},'InitialValueBuildCheck9',{{0,'OFF',[]}},'InitialValueBuildCheck10',{{0,'OFF',[]}},'InitialValueBuildCheck11',{{0,'OFF',[]}},'InitialValueBuildCheck12',{{0,'OFF',[]}},'InitialValueBuildCheck13',{{0,'OFF',[]}},'InitialValueBuildCheck14',{{0,'OFF',[]}},'InitialValueBuildCheck15',{{0,'OFF',[]}},'InitialValueBuildCheck16',{{0,'OFF',[]}},'TermValueBuildCheck1',{{0,'OFF',[]}},'TermValueBuildCheck2',{{0,'OFF',[]}},'TermValueBuildCheck3',{{0,'OFF',[]}},'TermValueBuildCheck4',{{0,'OFF',[]}},'TermValueBuildCheck5',{{0,'OFF',[]}},'TermValueBuildCheck6',{{0,'OFF',[]}},'TermValueBuildCheck7',{{0,'OFF',[]}},'TermValueBuildCheck8',{{0,'OFF',[]}},'TermValueBuildCheck9',{{0,'OFF',[]}},'TermValueBuildCheck10',{{0,'OFF',[]}},'TermValueBuildCheck11',{{0,'OFF',[]}},'TermValueBuildCheck12',{{0,'OFF',[]}},'TermValueBuildCheck13',{{0,'OFF',[]}},'TermValueBuildCheck14',{{0,'OFF',[]}},'TermValueBuildCheck15',{{0,'OFF',[]}},'TermValueBuildCheck16',{{0,'OFF',[]}})  RTISFcnParameters=struct('ChannelNo','int16','ChannelNumOf','int16','InitialValue1','double','InitialValue2','double','InitialValue3','double','InitialValue4','double','InitialValue5','double','InitialValue6','double','InitialValue7','double','InitialValue8','double','InitialValue9','double','InitialValue10','double','InitialValue11','double','InitialValue12','double','InitialValue13','double','InitialValue14','double','InitialValue15','double','InitialValue16','double','OutputMode','int16','TermValue1','double','TermValue2','double','TermValue3','double','TermValue4','double','TermValue5','double','TermValue6','double','TermValue7','double','TermValue8','double','TermValue9','double','TermValue10','double','TermValue11','double','TermValue12','double','TermValue13','double','TermValue14','double','TermValue15','double','TermValue16','double','EnableTermMode','int16','TLCFileName','char')  RTIBlockParaDefault=struct('ChannelNo',1,'ChannelNumOf',1,'InitialValue1',0,'InitialValue2',0,'InitialValue3',0,'InitialValue4',0,'InitialValue5',0,'InitialValue6',0,'InitialValue7',0,'InitialValue8',0,'InitialValue9',0,'InitialValue10',0,'InitialValue11',0,'InitialValue12',0,'InitialValue13',0,'InitialValue14',0,'InitialValue15',0,'InitialValue16',0,'OutputMode',ones(1,16),'TermValue1',0,'TermValue2',0,'TermValue3',0,'TermValue4',0,'TermValue5',0,'TermValue6',0,'TermValue7',0,'TermValue8',0,'TermValue9',0,'TermValue10',0,'TermValue11',0,'TermValue12',0,'TermValue13',0,'TermValue14',0,'TermValue15',0,'TermValue16',0,'EnableTermMode',0,'TLCFileName','rti120xdac_c1_dac','InitialValueBuildCheck1',0,'InitialValueBuildCheck2',0,'InitialValueBuildCheck3',0,'InitialValueBuildCheck4',0,'InitialValueBuildCheck5',0,'InitialValueBuildCheck6',0,'InitialValueBuildCheck7',0,'InitialValueBuildCheck8',0,'InitialValueBuildCheck9',0,'InitialValueBuildCheck10',0,'InitialValueBuildCheck11',0,'InitialValueBuildCheck12',0,'InitialValueBuildCheck13',0,'InitialValueBuildCheck14',0,'InitialValueBuildCheck15',0,'InitialValueBuildCheck16',0,'TermValueBuildCheck1',0,'TermValueBuildCheck2',0,'TermValueBuildCheck3',0,'TermValueBuildCheck4',0,'TermValueBuildCheck5',0,'TermValueBuildCheck6',0,'TermValueBuildCheck7',0,'TermValueBuildCheck8',0,'TermValueBuildCheck9',0,'TermValueBuildCheck10',0,'TermValueBuildCheck11',0,'TermValueBuildCheck12',0,'TermValueBuildCheck13',0,'TermValueBuildCheck14',0,'TermValueBuildCheck15',0,'TermValueBuildCheck16',0)
  DSPscale : Gain  Gain=1/10  SaturateOnIntegerOverflow=on  OutDataTypeStr=Inherit: Same as input  ParamDataTypeStr=Inherit: Same as input
  Saturation : Saturate  UpperLimit=3  LowerLimit=-3
  wires:
  Saturation/1 -> Current2V/1
  Current2V/1 -> DSPscale/1
  Motor current [A]/1 -> Saturation/1
  DSPscale/1 -> DAC_CLASS1_BL1/1

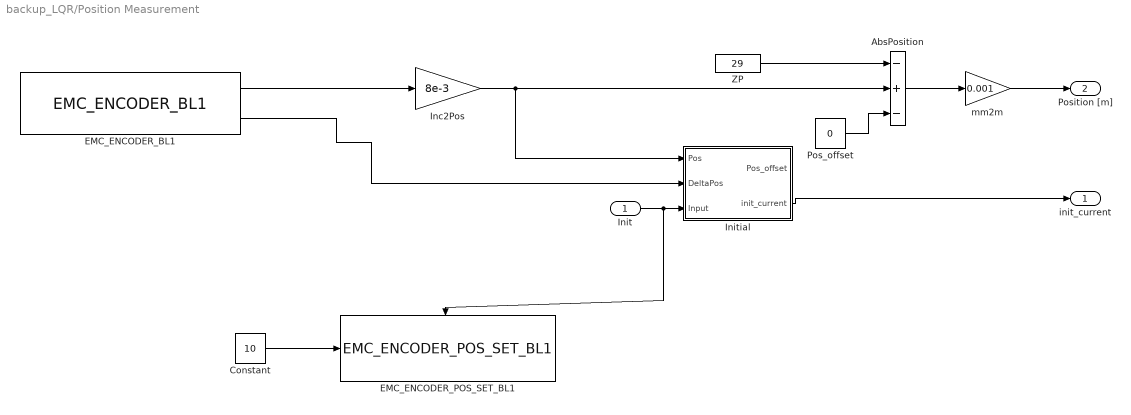
== system backup_LQR/Position Measurement ==
  Init : Inport
  AbsPosition : Sum  Inputs=-+-  SaturateOnIntegerOverflow=on
  Constant : Constant  Value=10
  EMC_ENCODER_BL1 : rtiemclib/EMC_ENCODER_BL1  DSProperties=struct('RTI',struct('Version',uint32(2),'BlockType',struct('isSLSource',uint8(1),'isSLSink',uint8(0),'isHWSource',uint8(1),'isHWSink',uint8(0),'isSetup',uint8(0),'isInline',uint8(1),'isNonInline',uint8(0),'isInterrupt',uint8(0),'isChannelwise',uint8(1)),'IOBoardType','DSEMC','UnitType','ENCODER','Identifier','ENCODER','DialogType','ML','BlockSet','RTIEMC','SlaveProcessor','NONE'))  RTIBlockInterface=struct('OutputPortsWidth',int32([1 1 1]),'OutputPortsActive',int32([1 1 0]),'OutputPortsName',{{'Position','Speed',['Index Detected']}},'OutputPortsDataType',{{'SS_DOUBLE','SS_DOUBLE','SS_BOOLEAN'}},'InitLevel',3,'IconTransparency','on','BlockDisplay',{{['EMC Encoder\nUnit: 1\nDIO class: 2\nPort: 1\nChannel: 1'],'center'}},'DialogFcn','rtiemcencodergui','BlockName',struct('Token',{{'EMC_ENCODER_BL1'}}))  RTIBlockParameters=struct('UnitNo',{{1,'OFF',[1 6]}},'DioClassNo',{{2,'OFF',[1 2]}},'PortNo',{{1,'OFF',[1 1]}},'ChannelNo',{{1,'OFF',[1 11]}},'HwSignalPin',{{['DIO1 ch1'],'OFF',[]}},'HwRefPin',{{'GND','OFF',[]}},'EnablePosMeasurement',{{1,'OFF',[0 1]}},'IndexSetMode',{{1,'OFF',[1 3]}},'EnableMinSpeed',{{0,'OFF',[0 1]}},'NumOfLines',{{'1024','OFF',[1 2097152]}},'InitAngleValue',{{'60','OFF',[0 359.99999]}},'IndexAngleValue',{{'0','OFF',[0 359.99999]}},'MinSpeedAngleValue',{{'45','OFF',[0.05 10000]}},'MinPosValue',{{'0','OFF',[-2097152 2097150.75]}},'MaxPosValue',{{'10000','OFF',[-2097151 2097151.75]}},'InitPosValue',{{'0','OFF',[-2097152 2097151.75]}},'IndexPosValue',{{'0','OFF',[-2097152 2097151.75]}},'MinSpeedPosValue',{{'100','OFF',[1 1000000]}},'IndexGateMode',{{0,'OFF',[0 1]}},'EnableNoiseFilter',{{0,'OFF',[0 1]}},'FilterInterval',{{'0','OFF',[0 0.01]}},'IndexDetectedOutPortMode',{{0,'OFF',[0 1]}},'BuildCheckAngleMeasurement',{{0,'OFF',[0 1]}},'BuildCheckAngleIndexMode',{{0,'OFF',[0 1]}},'BuildCheckPosIndexMode',{{0,'OFF',[0 1]}},'BuildCheckAngleMinSpeed',{{0,'OFF',[0 1]}},'BuildCheckPosMinSpeed',{{0,'OFF',[0 1]}},'TLCFileName',{{'rtiemcencoder','OFF',[]}})  RTISFcnParameters=struct('UnitNo','int32','DioClassNo','int32','PortNo','int32','ChannelNo','int32','EnablePosMeasurement','int32','IndexSetMode','int32','IndexDetectedOutPortMode','int32','EnableMinSpeed','int32','NumOfLines','uint32','InitAngleValue','double','IndexAngleValue','double','MinSpeedAngleValue','double','MinPosValue','double','MaxPosValue','double','InitPosValue','double','IndexPosValue','double','MinSpeedPosValue','double','IndexGateMode','int32','EnableNoiseFilter','int32','FilterInterval','double','TLCFileName','char')  RTIBlockParaDefault=struct('UnitNo',1,'DioClassNo',1,'PortNo',1,'ChannelNo',1,'HwSignalPin',['DIO1 ch1'],'HwRefPin','GND','EnablePosMeasurement',0,'IndexSetMode',1,'EnableMinSpeed',0,'NumOfLines',1024,'InitAngleValue',60,'IndexAngleValue',0,'MinSpeedAngleValue',45,'MinPosValue',0,'MaxPosValue',1023.75,'InitPosValue',0,'IndexPosValue',0,'MinSpeedPosValue',100,'IndexGateMode',0,'EnableNoiseFilter',0,'FilterInterval',0,'IndexDetectedOutPortMode',0,'BuildCheckAngleMeasurement',1,'BuildCheckAngleIndexMode',0,'BuildCheckPosIndexMode',0,'BuildCheckAngleMinSpeed',0,'BuildCheckPosMinSpeed',0,'TLCFileName','rtiemcencoder')
      settings: SourceProductName=dSPACE RTI Electric Motor Control Blockset
  EMC_ENCODER_POS_SET_BL1 : rtiemclib/EMC_ENCODER_POS_SET_BL1  DSProperties=struct('RTI',struct('Version',uint32(1),'BlockType',struct('isSLSource',uint8(0),'isSLSink',uint8(1),'isHWSource',uint8(0),'isHWSink',uint8(1),'isSetup',uint8(0),'isInline',uint8(1),'isNonInline',uint8(0),'isInterrupt',uint8(0),'isChannelwise',uint8(1)),'IOBoardType','DSEMC','UnitType','ENCODER','Identifier','ENCODERPOSSET','DialogType','ML','BlockSet','RTIEMC','SlaveProcessor','NONE'))  RTIBlockInterface=struct('InputPortsWidth',int32(1),'InputPortsActive',1,'InputPortsDataType',{{'SS_DOUBLE'}},'InputPortsName',{{'Position'}},'TriggerPort',{{'rising'}},'InitLevel',3,'IconTransparency','on','BlockDisplay',{{['EMC Encoder Position Set\nUnit: 1\nDIO class: 2\nPort: 1\nChannel: 1'],'center'}},'DialogFcn','rtiemcencoderpossetgui','BlockName',struct('Token',{{'EMC_ENCODER_POS_SET_BL1'}}))  RTIBlockParameters=struct('EncoderIdIndex',{{2,'OFF',[1 4]}},'UnitNo',{{1,'OFF',[]}},'DioClassNo',{{2,'OFF',[]}},'PortNo',{{1,'OFF',[]}},'ChannelNo',{{1,'OFF',[]}},'EnablePosMeasurement',{{1,'OFF',[]}},'NumOfLines',{{1024,'OFF',[]}},'TLCFileName',{{'rtiemcencoderposset','OFF',[]}})  RTISFcnParameters=struct('EncoderIdIndex','int32','UnitNo','int32','DioClassNo','int32','PortNo','int32','ChannelNo','int32','EnablePosMeasurement','int32','NumOfLines','int32','TLCFileName','char')  RTIBlockParaDefault=struct('EncoderIdIndex',1,'UnitNo',-1,'DioClassNo',-1,'PortNo',-1,'ChannelNo',-1,'EnablePosMeasurement',0,'NumOfLines',1024,'TLCFileName','rtiemcencoderposset')
      settings: SourceProductName=dSPACE RTI Electric Motor Control Blockset
  Inc2Pos : Gain  Gain=8e-3  SaturateOnIntegerOverflow=on  OutDataTypeStr=Inherit: Same as input  ParamDataTypeStr=Inherit: Same as input
  Initial : Subsystem
  Pos_offset : Constant  Value=0
  ZP : Constant  Value=29
  mm2m : Gain  Gain=0.001
  init_current : Outport  VectorParamsAs1DForOutWhenUnconnected=off
  Position [m] : Outport  Port=2  VectorParamsAs1DForOutWhenUnconnected=off
  wires:
  AbsPosition/1 -> mm2m/1
  Inc2Pos/1 -> Initial/1(Pos), AbsPosition/2
  Initial/2(init_current) -> init_current/1
  mm2m/1 -> Position [m]/1
  EMC_ENCODER_BL1/2 -> Initial/2(DeltaPos)
  ZP/1 -> AbsPosition/1
  Init/1 -> Initial/3(Input), EMC_ENCODER_POS_SET_BL1/Trigger
  Constant/1 -> EMC_ENCODER_POS_SET_BL1/1
  Pos_offset/1 -> AbsPosition/3
  EMC_ENCODER_BL1/1 -> Inc2Pos/1
